simulink model "lup"  (Simulink 5.0)
settings: Solver=ode45  StartTime=0.0  StopTime=10.0  RelTol=1e-3
undefined symbols (not defined in the file or in its folder): matricaA, vektorb
libraries: dspsrcs4 x2, dspfactors x1, dspsolvers x1
settings Model: LastModifiedBy=yeti

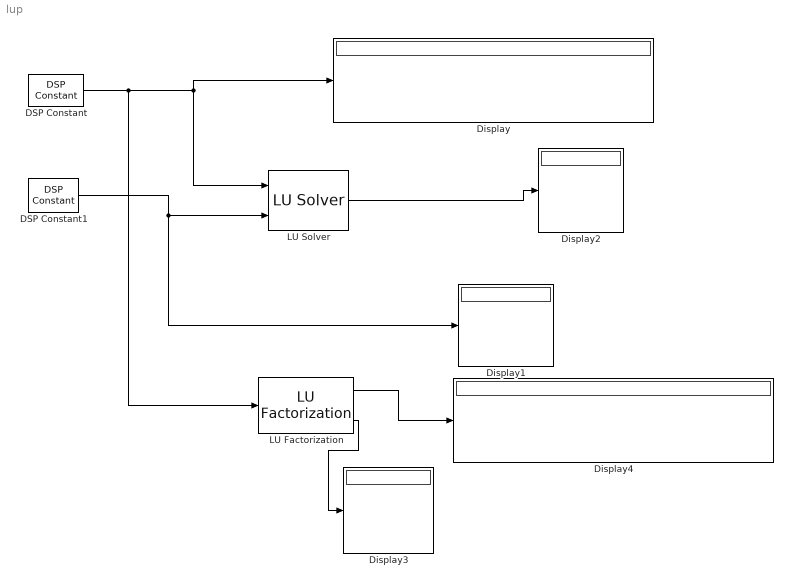
== system lup ==
  DSP Constant : dspsrcs4/DSP Constant  Value=matricaA  SampleMode=Discrete  discreteOutput=Sample-based  continuousOutput=Sample-based  sampTime=1  framePeriod=2  dataType=Inherit from 'Constant value'  wordLen=16  udDataType=sfix(16)  fracBitsMode=Best precision  numFracBits=15  InterpretAs1D=-inf  Ts=-inf  FramebasedOutput=-inf
  DSP Constant1 : dspsrcs4/DSP Constant  Value=vektorb  SampleMode=Discrete  discreteOutput=Sample-based  continuousOutput=Sample-based  sampTime=1  framePeriod=2  dataType=Inherit from 'Constant value'  wordLen=16  udDataType=sfix(16)  fracBitsMode=Best precision  numFracBits=15  InterpretAs1D=-inf  Ts=-inf  FramebasedOutput=-inf
  Display{,1..4} (5 alike) : Display
  LU Factorization : dspfactors/LU Factorization  singular=off
  LU Solver : dspsolvers/LU Solver
  wires:
  DSP Constant/1 -> Display/1, LU Solver/1, LU Factorization/1
  DSP Constant1/1 -> LU Solver/2, Display1/1
  LU Solver/1 -> Display2/1
  LU Factorization/2 -> Display3/1
  LU Factorization/1 -> Display4/1
